simulink model "Copy_of_cd_barrowman_method"  (R2023a)
settings: Solver=VariableStepAuto  StartTime=0.0  StopTime=10.0  RelTol=1e-3
settings Model: Creator=aleco  LastModifiedBy=aleco

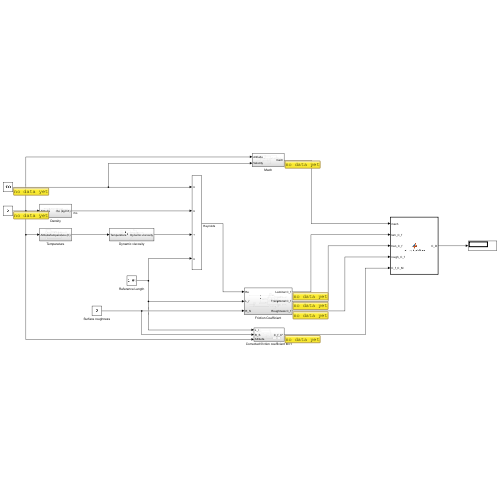
[thumbnail: Simulink's stored preview of the top-level diagram]
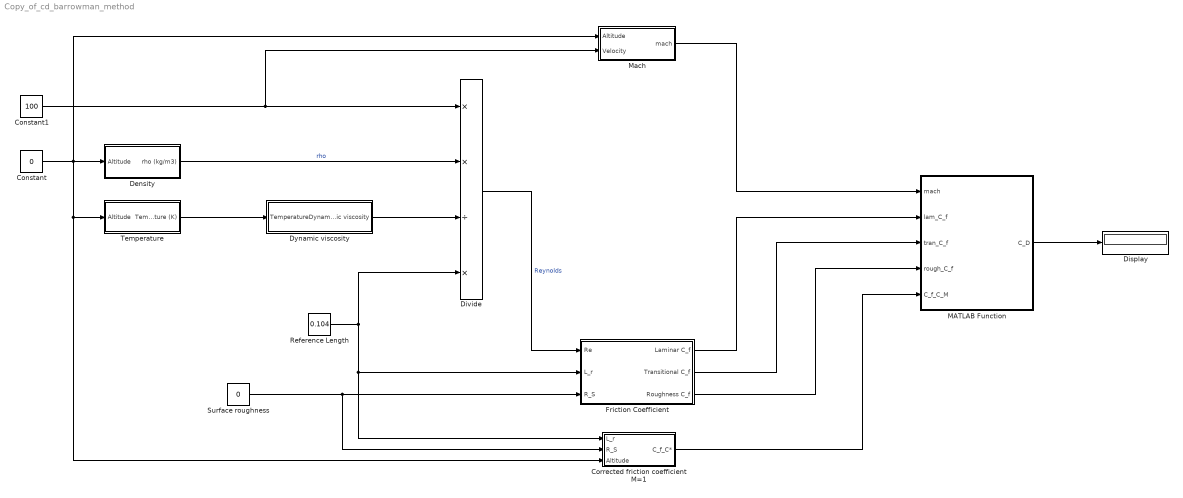
== system Copy_of_cd_barrowman_method ==
  Constant : Constant  Value=0
  Constant1 : Constant  Value=100
  Corrected friction coefficient M=1 : Subsystem
  Density : Subsystem
  Display : Display
  Divide : Product  Inputs=**/*
  Dynamic viscosity : Subsystem
  Friction Coefficient : Subsystem
  MATLAB Function : MATLAB Function  TreatAsAtomicUnit=on
  Mach : Subsystem
  Reference Length : Constant  Value=0.104
  Surface roughness : Constant  Value=0
  Temperature : Subsystem
  wires:
  Constant1/1 -> Divide/1, Mach/2(Velocity)
  Temperature/1(Temperature (K)) -> Dynamic viscosity/1(Temperature)
  Density/1(rho (kg/m3)) -> Divide/2  "rho"
  Reference Length/1 -> Divide/4, Corrected friction coefficient M=1/1(L_r), Friction Coefficient/2(L_r)
  Dynamic viscosity/1(Dynamic viscosity) -> Divide/3
  Surface roughness/1 -> Friction Coefficient/3(R_S), Corrected friction coefficient M=1/2(R_S)
  Divide/1 -> Friction Coefficient/1(Re)  "Reynolds"
  Constant/1 -> Mach/1(Altitude), Corrected friction coefficient M=1/3(Altitude), Temperature/1(Altitude), Density/1(Altitude)
  Mach/1(mach) -> MATLAB Function/1(mach)
  Friction Coefficient/1(Laminar C_f) -> MATLAB Function/2(lam_C_f)
  Friction Coefficient/2(Transitional C_f) -> MATLAB Function/3(tran_C_f)
  Friction Coefficient/3(Roughness C_f) -> MATLAB Function/4(rough_C_f)
  Corrected friction coefficient M=1/1(C_f_C*) -> MATLAB Function/5(C_f_C_M)
  MATLAB Function/1(C_D) -> Display/1

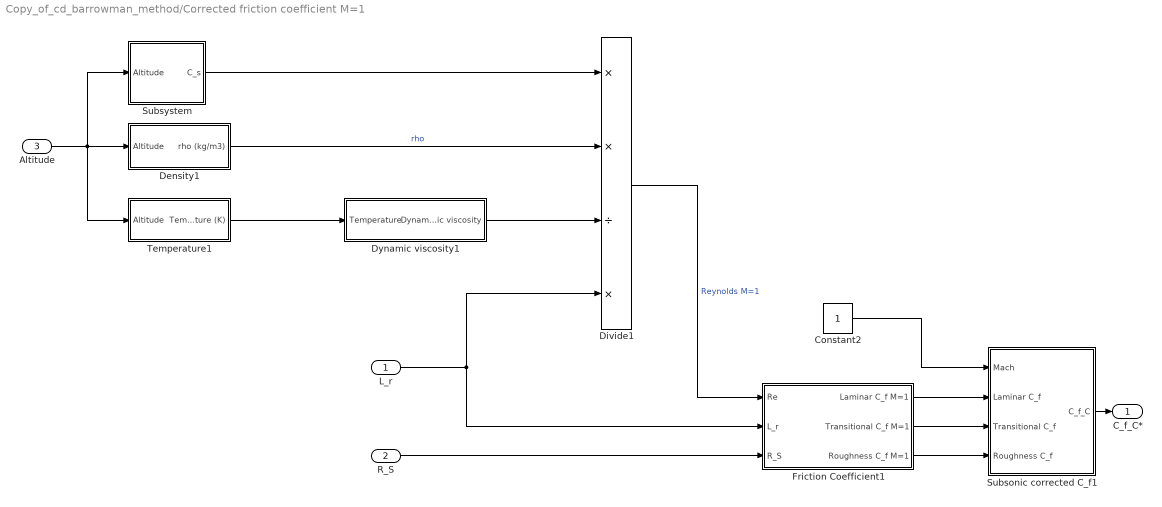
== system Copy_of_cd_barrowman_method/Corrected friction coefficient M=1 ==
  L_r : Inport
  R_S : Inport  Port=2
  Altitude : Inport  Port=3
  Constant2 : Constant
  Density1 : Subsystem
  Divide1 : Product  Inputs=**/*
  Dynamic viscosity1 : Subsystem
  Friction Coefficient1 : Subsystem
  Subsonic corrected C_f1 : Subsystem
  Subsystem : Subsystem
  Temperature1 : Subsystem
  C_f_C* : Outport
  wires:
  Temperature1/1(Temperature (K)) -> Dynamic viscosity1/1(Temperature)
  Subsystem/1(C_s) -> Divide1/1
  Divide1/1 -> Friction Coefficient1/1(Re)  "Reynolds M=1"
  R_S/1 -> Friction Coefficient1/3(R_S)
  Friction Coefficient1/1(Laminar C_f M=1) -> Subsonic corrected C_f1/2(Laminar C_f)
  L_r/1 -> Divide1/4, Friction Coefficient1/2(L_r)
  Friction Coefficient1/2(Transitional C_f M=1) -> Subsonic corrected C_f1/3(Transitional C_f)
  Friction Coefficient1/3(Roughness C_f M=1) -> Subsonic corrected C_f1/4(Roughness C_f)
  Dynamic viscosity1/1(Dynamic viscosity) -> Divide1/3
  Constant2/1 -> Subsonic corrected C_f1/1(Mach)
  Altitude/1 -> Subsystem/1(Altitude), Temperature1/1(Altitude), Density1/1(Altitude)
  Density1/1(rho (kg/m3)) -> Divide1/2  "rho"
  Subsonic corrected C_f1/1(C_f_C) -> C_f_C*/1

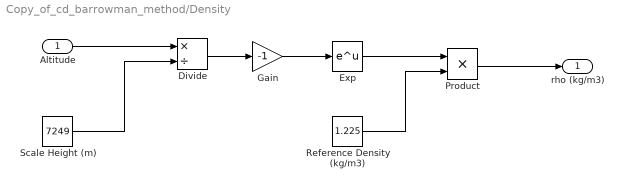
== system Copy_of_cd_barrowman_method/Density ==
  Altitude : Inport
  Divide : Product  Inputs=*/
  Exp : Math
  Gain : Gain  Gain=-1
  Product : Product
  Reference Density (kg/m3) : Constant  Value=1.225
  Scale Height (m) : Constant  Value=7249
  rho (kg/m3) : Outport
  wires:
  Altitude/1 -> Divide/1
  Scale Height (m)/1 -> Divide/2
  Divide/1 -> Gain/1
  Gain/1 -> Exp/1
  Exp/1 -> Product/1
  Reference Density (kg/m3)/1 -> Product/2
  Product/1 -> rho (kg/m3)/1

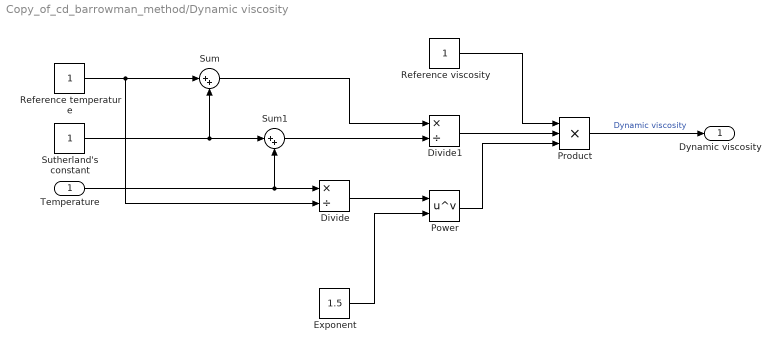
== system Copy_of_cd_barrowman_method/Dynamic viscosity ==
  Temperature : Inport
  Divide : Product  Inputs=*/
  Divide1 : Product  Inputs=*/
  Exponent : Constant  Value=1.5
  Power : Math  Operator=pow
  Product : Product  Inputs=3
  Reference temperature : Constant
  Reference viscosity : Constant
  Sum : Sum  Inputs=|++
  Sum1 : Sum  Inputs=|++
  Sutherland's constant : Constant
  Dynamic viscosity : Outport
  wires:
  Sum/1 -> Divide1/1
  Divide/1 -> Power/1
  Temperature/1 -> Sum1/2, Divide/1
  Sutherland's constant/1 -> Sum/2, Sum1/1
  Reference temperature/1 -> Divide/2, Sum/1
  Sum1/1 -> Divide1/2
  Exponent/1 -> Power/2
  Divide1/1 -> Product/2
  Product/1 -> Dynamic viscosity/1  "Dynamic viscosity"
  Reference viscosity/1 -> Product/1
  Power/1 -> Product/3

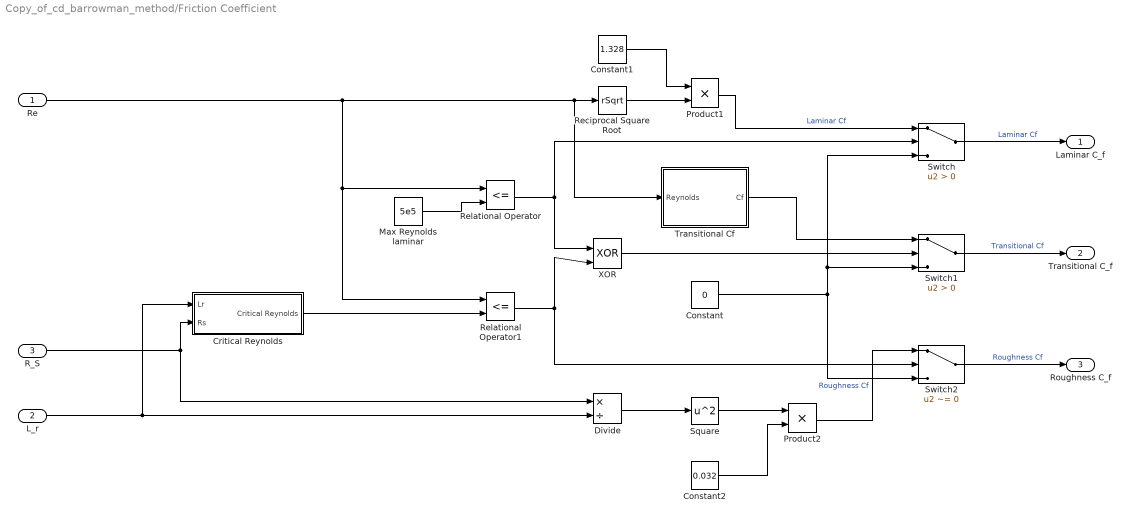
== system Copy_of_cd_barrowman_method/Friction Coefficient ==
  Re : Inport
  L_r : Inport  Port=2
  R_S : Inport  Port=3
  Constant : Constant  Value=0
  Constant1 : Constant  Value=1.328
  Constant2 : Constant  Value=0.032
  Critical Reynolds : Subsystem
  Divide : Product  Inputs=*/
  Max Reynolds laminar : Constant  Value=5e5
  Product1 : Product
  Product2 : Product
  Reciprocal Square Root : Sqrt  Operator=rSqrt
  Relational Operator : RelationalOperator  Operator=<=  OutDataTypeStr=boolean  RndMeth=Simplest  InputSameDT=off
  Relational Operator1 : RelationalOperator  Operator=<=  OutDataTypeStr=boolean  RndMeth=Simplest  InputSameDT=off
  Square : Math  Operator=square
  Switch : Switch  Criteria=u2 > Threshold  SaturateOnIntegerOverflow=off  InputSameDT=off
  Switch1 : Switch  Criteria=u2 > Threshold  SaturateOnIntegerOverflow=off  InputSameDT=off
  Switch2 : Switch  Criteria=u2 ~= 0  SaturateOnIntegerOverflow=off  InputSameDT=off
  Transitional Cf : Subsystem
  XOR : Logic  Operator=XOR  IconShape=distinctive  AllPortsSameDT=off  OutDataTypeStr=boolean
  Laminar C_f : Outport
  Transitional C_f : Outport  Port=2
  Roughness C_f : Outport  Port=3
  wires:
  Constant/1 -> Switch/3, Switch1/3, Switch2/3
  Reciprocal Square Root/1 -> Product1/2
  Transitional Cf/1(Cf) -> Switch1/1
  Switch2/1 -> Roughness C_f/1  "Roughness Cf"
  Product1/1 -> Switch/1  "Laminar Cf"
  Critical Reynolds/1(Critical Reynolds) -> Relational Operator1/2
  Relational Operator1/1 -> Switch2/2, XOR/2
  Re/1 -> Transitional Cf/1(Reynolds), Reciprocal Square Root/1, Relational Operator/1, Relational Operator1/1
  Product2/1 -> Switch2/1  "Roughness Cf"
  XOR/1 -> Switch1/2
  R_S/1 -> Critical Reynolds/2(Rs), Divide/1
  Constant1/1 -> Product1/1
  Switch1/1 -> Transitional C_f/1  "Transitional Cf"
  L_r/1 -> Critical Reynolds/1(Lr), Divide/2
  Relational Operator/1 -> Switch/2, XOR/1
  Max Reynolds laminar/1 -> Relational Operator/2
  Divide/1 -> Square/1
  Switch/1 -> Laminar C_f/1  "Laminar Cf"
  Square/1 -> Product2/1
  Constant2/1 -> Product2/2

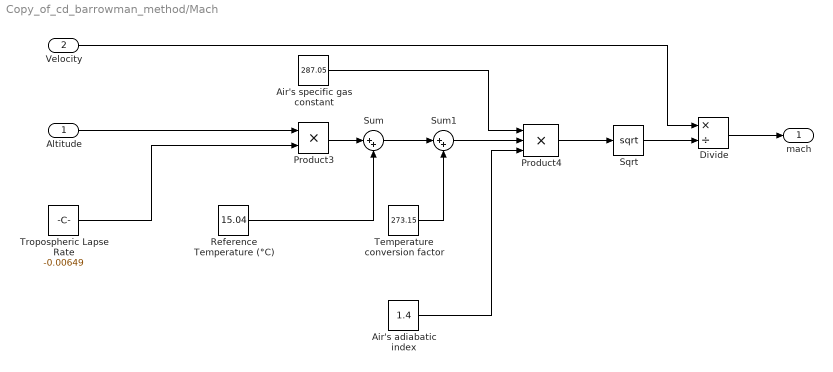
== system Copy_of_cd_barrowman_method/Mach ==
  Altitude : Inport
  Velocity : Inport  Port=2
  Air's adiabatic index : Constant  Value=1.4
  Air's specific gas constant : Constant  Value=287.05
  Divide : Product  Inputs=*/
  Product3 : Product
  Product4 : Product  Inputs=3
  Reference Temperature (°C) : Constant  Value=15.04
  Sqrt : Sqrt
  Sum : Sum  Inputs=|++
  Sum1 : Sum  Inputs=|++
  Temperature conversion factor : Constant  Value=273.15
  Tropospheric Lapse Rate : Constant  Value=-0.00649
  mach : Outport
  wires:
  Product4/1 -> Sqrt/1
  Product3/1 -> Sum/1
  Air's adiabatic index/1 -> Product4/3
  Tropospheric Lapse Rate/1 -> Product3/2
  Air's specific gas constant/1 -> Product4/1
  Sum/1 -> Sum1/1
  Reference Temperature (°C)/1 -> Sum/2
  Altitude/1 -> Product3/1
  Velocity/1 -> Divide/1
  Divide/1 -> mach/1
  Temperature conversion factor/1 -> Sum1/2
  Sum1/1 -> Product4/2
  Sqrt/1 -> Divide/2

== system Copy_of_cd_barrowman_method/Temperature ==
  Altitude : Inport
  Factor of conversion to K : Constant  Value=273.15
  Product3 : Product
  Reference Temperature (°C) : Constant  Value=15.04
  Sum : Sum  Inputs=|++
  Sum1 : Sum  Inputs=|++
  Tropospheric Lapse Rate : Constant  Value=-0.00649
  Temperature (K) : Outport
  wires:
  Altitude/1 -> Product3/1
  Sum/1 -> Sum1/1
  Tropospheric Lapse Rate/1 -> Product3/2
  Product3/1 -> Sum/1
  Factor of conversion to K/1 -> Sum1/2
  Sum1/1 -> Temperature (K)/1
  Reference Temperature (°C)/1 -> Sum/2

== system Copy_of_cd_barrowman_method/Corrected friction coefficient M=1/Density1 ==
  Altitude : Inport
  Divide : Product  Inputs=*/
  Exp : Math
  Gain : Gain  Gain=-1
  Product : Product
  Reference Density (kg/m3) : Constant  Value=1.225
  Scale Height (m) : Constant  Value=7249
  rho (kg/m3) : Outport
  wires:
  Altitude/1 -> Divide/1
  Scale Height (m)/1 -> Divide/2
  Divide/1 -> Gain/1
  Gain/1 -> Exp/1
  Exp/1 -> Product/1
  Reference Density (kg/m3)/1 -> Product/2
  Product/1 -> rho (kg/m3)/1

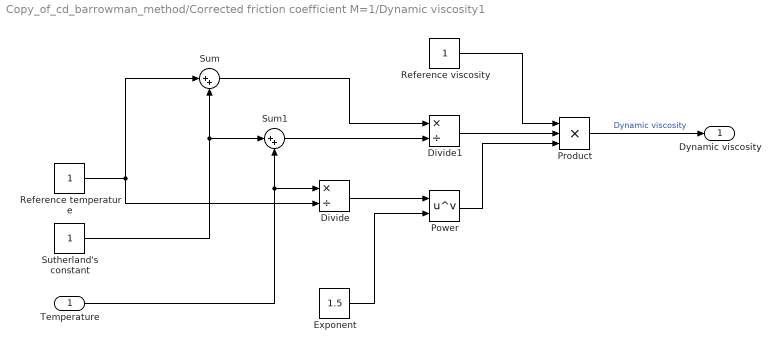
== system Copy_of_cd_barrowman_method/Corrected friction coefficient M=1/Dynamic viscosity1 ==
  Temperature : Inport
  Divide : Product  Inputs=*/
  Divide1 : Product  Inputs=*/
  Exponent : Constant  Value=1.5
  Power : Math  Operator=pow
  Product : Product  Inputs=3
  Reference temperature : Constant
  Reference viscosity : Constant
  Sum : Sum  Inputs=|++
  Sum1 : Sum  Inputs=|++
  Sutherland's constant : Constant
  Dynamic viscosity : Outport
  wires:
  Sum/1 -> Divide1/1
  Divide/1 -> Power/1
  Temperature/1 -> Sum1/2, Divide/1
  Sutherland's constant/1 -> Sum/2, Sum1/1
  Reference temperature/1 -> Divide/2, Sum/1
  Sum1/1 -> Divide1/2
  Exponent/1 -> Power/2
  Divide1/1 -> Product/2
  Product/1 -> Dynamic viscosity/1  "Dynamic viscosity"
  Reference viscosity/1 -> Product/1
  Power/1 -> Product/3

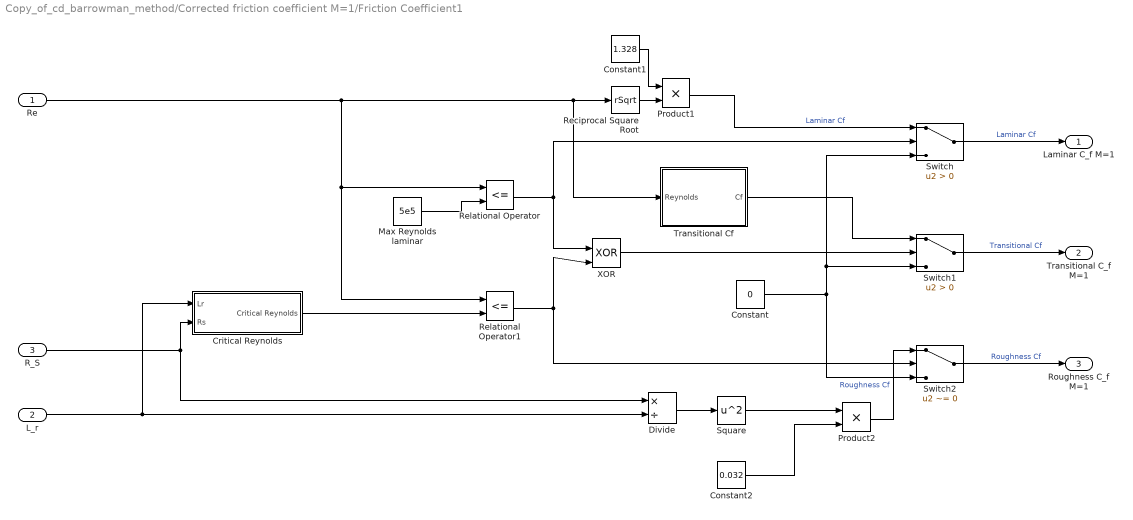
== system Copy_of_cd_barrowman_method/Corrected friction coefficient M=1/Friction Coefficient1 ==
  Re : Inport
  L_r : Inport  Port=2
  R_S : Inport  Port=3
  Constant : Constant  Value=0
  Constant1 : Constant  Value=1.328
  Constant2 : Constant  Value=0.032
  Critical Reynolds : Subsystem
  Divide : Product  Inputs=*/
  Max Reynolds laminar : Constant  Value=5e5
  Product1 : Product
  Product2 : Product
  Reciprocal Square Root : Sqrt  Operator=rSqrt
  Relational Operator : RelationalOperator  Operator=<=  OutDataTypeStr=boolean  RndMeth=Simplest  InputSameDT=off
  Relational Operator1 : RelationalOperator  Operator=<=  OutDataTypeStr=boolean  RndMeth=Simplest  InputSameDT=off
  Square : Math  Operator=square
  Switch : Switch  Criteria=u2 > Threshold  SaturateOnIntegerOverflow=off  InputSameDT=off
  Switch1 : Switch  Criteria=u2 > Threshold  SaturateOnIntegerOverflow=off  InputSameDT=off
  Switch2 : Switch  Criteria=u2 ~= 0  SaturateOnIntegerOverflow=off  InputSameDT=off
  Transitional Cf : Subsystem
  XOR : Logic  Operator=XOR  IconShape=distinctive  AllPortsSameDT=off  OutDataTypeStr=boolean
  Laminar C_f M=1 : Outport
  Transitional C_f M=1 : Outport  Port=2
  Roughness C_f M=1 : Outport  Port=3
  wires:
  Constant/1 -> Switch/3, Switch1/3, Switch2/3
  Reciprocal Square Root/1 -> Product1/2
  Transitional Cf/1(Cf) -> Switch1/1
  Switch2/1 -> Roughness C_f M=1/1  "Roughness Cf"
  Product1/1 -> Switch/1  "Laminar Cf"
  Critical Reynolds/1(Critical Reynolds) -> Relational Operator1/2
  Relational Operator1/1 -> Switch2/2, XOR/2
  Re/1 -> Transitional Cf/1(Reynolds), Reciprocal Square Root/1, Relational Operator/1, Relational Operator1/1
  Product2/1 -> Switch2/1  "Roughness Cf"
  XOR/1 -> Switch1/2
  R_S/1 -> Critical Reynolds/2(Rs), Divide/1
  Constant1/1 -> Product1/1
  Switch1/1 -> Transitional C_f M=1/1  "Transitional Cf"
  L_r/1 -> Critical Reynolds/1(Lr), Divide/2
  Relational Operator/1 -> Switch/2, XOR/1
  Max Reynolds laminar/1 -> Relational Operator/2
  Divide/1 -> Square/1
  Switch/1 -> Laminar C_f M=1/1  "Laminar Cf"
  Square/1 -> Product2/1
  Constant2/1 -> Product2/2

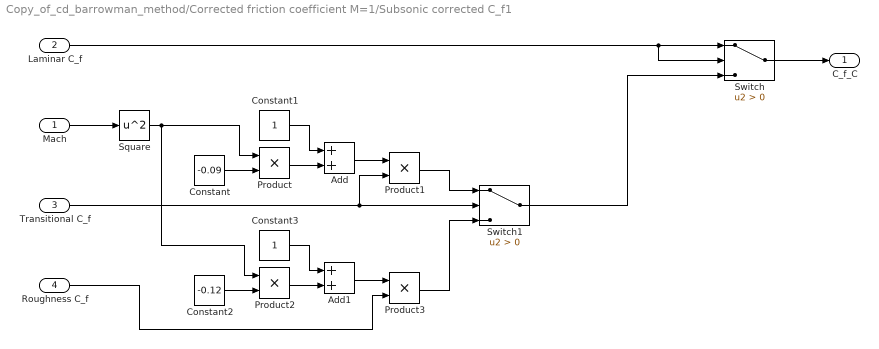
== system Copy_of_cd_barrowman_method/Corrected friction coefficient M=1/Subsonic corrected C_f1 ==
  Mach : Inport
  Laminar C_f : Inport  Port=2
  Transitional C_f : Inport  Port=3
  Roughness C_f : Inport  Port=4
  Add : Sum
  Add1 : Sum
  Constant : Constant  Value=-0.09
  Constant1 : Constant
  Constant2 : Constant  Value=-0.12
  Constant3 : Constant
  Product{,1..3} (4 alike) : Product
  Square : Math  Operator=square
  Switch : Switch  Criteria=u2 > Threshold  SaturateOnIntegerOverflow=off  InputSameDT=off
  Switch1 : Switch  Criteria=u2 > Threshold  SaturateOnIntegerOverflow=off  InputSameDT=off
  C_f_C : Outport
  wires:
  Laminar C_f/1 -> Switch/2, Switch/1
  Switch/1 -> C_f_C/1
  Transitional C_f/1 -> Product1/2, Switch1/2
  Mach/1 -> Square/1
  Constant/1 -> Product/2
  Square/1 -> Product2/1, Product/1
  Constant1/1 -> Add/1
  Product/1 -> Add/2
  Add/1 -> Product1/1
  Product1/1 -> Switch1/1
  Switch1/1 -> Switch/3
  Constant2/1 -> Product2/2
  Add1/1 -> Product3/1
  Product2/1 -> Add1/2
  Constant3/1 -> Add1/1
  Roughness C_f/1 -> Product3/2
  Product3/1 -> Switch1/3

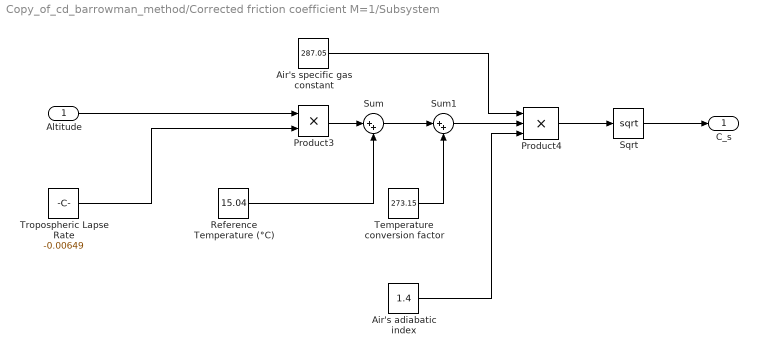
== system Copy_of_cd_barrowman_method/Corrected friction coefficient M=1/Subsystem ==
  Altitude : Inport
  Air's adiabatic index : Constant  Value=1.4
  Air's specific gas constant : Constant  Value=287.05
  Product3 : Product
  Product4 : Product  Inputs=3
  Reference Temperature (°C) : Constant  Value=15.04
  Sqrt : Sqrt
  Sum : Sum  Inputs=|++
  Sum1 : Sum  Inputs=|++
  Temperature conversion factor : Constant  Value=273.15
  Tropospheric Lapse Rate : Constant  Value=-0.00649
  C_s : Outport
  wires:
  Sum/1 -> Sum1/1
  Air's specific gas constant/1 -> Product4/1
  Air's adiabatic index/1 -> Product4/3
  Sum1/1 -> Product4/2
  Product4/1 -> Sqrt/1
  Temperature conversion factor/1 -> Sum1/2
  Tropospheric Lapse Rate/1 -> Product3/2
  Product3/1 -> Sum/1
  Reference Temperature (°C)/1 -> Sum/2
  Altitude/1 -> Product3/1
  Sqrt/1 -> C_s/1

== system Copy_of_cd_barrowman_method/Corrected friction coefficient M=1/Temperature1 ==
  Altitude : Inport
  Factor of conversion to K : Constant  Value=273.15
  Product3 : Product
  Reference Temperature (°C) : Constant  Value=15.04
  Sum : Sum  Inputs=|++
  Sum1 : Sum  Inputs=|++
  Tropospheric Lapse Rate : Constant  Value=-0.00649
  Temperature (K) : Outport
  wires:
  Altitude/1 -> Product3/1
  Sum/1 -> Sum1/1
  Tropospheric Lapse Rate/1 -> Product3/2
  Product3/1 -> Sum/1
  Factor of conversion to K/1 -> Sum1/2
  Sum1/1 -> Temperature (K)/1
  Reference Temperature (°C)/1 -> Sum/2

== system Copy_of_cd_barrowman_method/Friction Coefficient/Critical Reynolds ==
  Lr : Inport
  Rs : Inport  Port=2
  Constant : Constant  Value=51
  Constant1 : Constant  Value=-1.039
  Divide : Product  Inputs=*/
  Power : Math  Operator=pow
  Product1 : Product
  Critical Reynolds : Outport
  wires:
  Divide/1 -> Power/1
  Power/1 -> Product1/1
  Constant1/1 -> Power/2
  Constant/1 -> Product1/2
  Product1/1 -> Critical Reynolds/1  "Critical Reynolds"
  Lr/1 -> Divide/2
  Rs/1 -> Divide/1

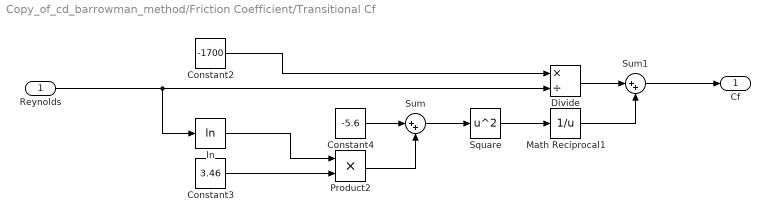
== system Copy_of_cd_barrowman_method/Friction Coefficient/Transitional Cf ==
  Reynolds : Inport
  Constant2 : Constant  Value=-1700
  Constant3 : Constant  Value=3.46
  Constant4 : Constant  Value=-5.6
  Divide : Product  Inputs=*/
  Math Reciprocal1 : Math  Operator=reciprocal  SignedPower=on
  Product2 : Product
  Square : Math  Operator=square
  Sum : Sum  Inputs=|++
  Sum1 : Sum  Inputs=|++
  ln : Math  Operator=log
  Cf : Outport
  wires:
  Math Reciprocal1/1 -> Sum1/2
  Constant2/1 -> Divide/1
  Product2/1 -> Sum/2
  Reynolds/1 -> ln/1, Divide/2
  Square/1 -> Math Reciprocal1/1
  Constant4/1 -> Sum/1
  Divide/1 -> Sum1/1
  ln/1 -> Product2/1
  Constant3/1 -> Product2/2
  Sum/1 -> Square/1
  Sum1/1 -> Cf/1

== system Copy_of_cd_barrowman_method/Corrected friction coefficient M=1/Friction Coefficient1/Critical Reynolds ==
  Lr : Inport
  Rs : Inport  Port=2
  Constant : Constant  Value=51
  Constant1 : Constant  Value=-1.039
  Divide : Product  Inputs=*/
  Power : Math  Operator=pow
  Product1 : Product
  Critical Reynolds : Outport
  wires:
  Divide/1 -> Power/1
  Power/1 -> Product1/1
  Constant1/1 -> Power/2
  Constant/1 -> Product1/2
  Product1/1 -> Critical Reynolds/1  "Critical Reynolds"
  Lr/1 -> Divide/2
  Rs/1 -> Divide/1

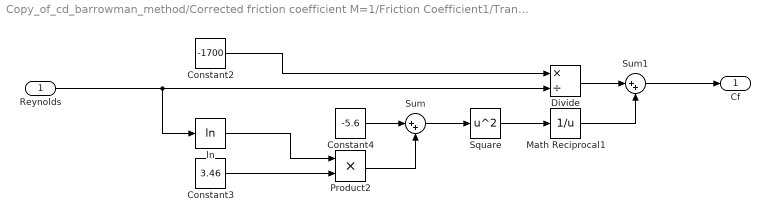
== system Copy_of_cd_barrowman_method/Corrected friction coefficient M=1/Friction Coefficient1/Transitional Cf ==
  Reynolds : Inport
  Constant2 : Constant  Value=-1700
  Constant3 : Constant  Value=3.46
  Constant4 : Constant  Value=-5.6
  Divide : Product  Inputs=*/
  Math Reciprocal1 : Math  Operator=reciprocal  SignedPower=on
  Product2 : Product
  Square : Math  Operator=square
  Sum : Sum  Inputs=|++
  Sum1 : Sum  Inputs=|++
  ln : Math  Operator=log
  Cf : Outport
  wires:
  Math Reciprocal1/1 -> Sum1/2
  Constant2/1 -> Divide/1
  Product2/1 -> Sum/2
  Reynolds/1 -> ln/1, Divide/2
  Square/1 -> Math Reciprocal1/1
  Constant4/1 -> Sum/1
  Divide/1 -> Sum1/1
  ln/1 -> Product2/1
  Constant3/1 -> Product2/2
  Sum/1 -> Square/1
  Sum1/1 -> Cf/1

== matlab function Copy_of_cd_barrowman_method/MATLAB Function ==
  data: mach input; C_D output; lam_C_f input; tran_C_f input; rough_C_f input; C_f_C_M input
function C_D = cd_calculation(mach,lam_C_f,tran_C_f,rough_C_f,C_f_C_M)
% %% SETUP OF THE ROCKET'S GEOMETRY
% N = 4; % number of fins
% A_T = 0.0135; % planform area of a single fin
% A_r = 0.008495; % reference area
% f_b = 20.77; % fineness ratio of the body
% A_W_B = 1.245; % total wetted area of the body
% S = 0.1; % fin's span
% gamma_L = pi/4; % leading edge sweepback angle
% r_L = 0.002; % radius of the rounded leading edge
% c_r = 0.2; % fin's root chord
% h_r = 0.004; % root trailing edge thickness of the fin
% t_r = 0.05; % maximum thickness of the fin
% gamma_C = 0.994; % midcord line sweepback angle
% A_B_f = 9e-3; % fin's base area
% f_n = 5; % fineness ratio of the nose
% A_B = 0.008495; % base area
% %% C_D CALCULATION
% if mach^2 <= 0.1 %incompressible flow
%     %% COEFFICIENT OF FRICTION
%     C_f = lam_C_f + tran_C_f + rough_C_f; % adding the C_f directly as just
%     % one of them will be different than zero
%     %% FRICTION DRAG COEFFICIENT
%     C_D_f_t = 2 * N * C_f * A_T * A_r; % tail
%     C_D_f_b = (1 + (0.5 / f_b)) * C_f * A_W_B / A_r; % body
%     C_D_f = C_D_f_b + C_D_f_t; % friction drag coefficient
%     %% FINS' DRAG COEFFICIENTS
%     delta_C_D = ((1 - mach^2)^-0.417) - 1;
%     C_D_L_T = 2 * N * S * r_L * cos(gamma_L)^2 * delta_C_D / A_r; % leading
%     % edge pressure drag
%     C_f_B = 2 * C_f * c_r / h_r;
%     C_D_B_T = 0.135 * N / (C_f_B^(1/3)); % trailing edge base drag
%     AR = S^2 / A_T; % aspect ratio of the fin
%     epsilon = AR * t_r^(1/3) / c_r;
%     C_D_TT_M = 1.15 * (t_r / c_r)^(5/3) * (1.61 + epsilon - ...
%         sqrt((epsilon - 1.43)^2 + 0.578));
%     K = cos(gamma_C)^2 + ((C_D_TT_M * A_r / (C_f_C_M * A_T) - ...
%         4 * t_r * cos(gamma_C) / c_r) / ...
%         (120 * (t_r / c_r)^4 * cos(gamma_C)^2));% prandtl correcting factor
%     C_D_TT = 4 * N * C_f * (A_T / A_r) * (t_r * cos(gamma_C) / c_r + ...
%         30 * (t_r / c_r)^4 * cos(gamma_C)^2 / ...
%         ((K - mach^2 * cos(gamma_C)^2)^(3/2)));% thickness pressure drag
%     % coefficient
%     %% BODY'S DRAG COEFFICIENTS
%     K_og = 1 + (6.82 * A_W_B * C_f_C_M * (f_n + 1)^2.22 / (f_b^3 * A_r));
%     % ogive
%     C_D_P = 6 * A_W_B * C_f / (f_b^3 * A_r * (K_og - mach^2)^0.6);% body
%     % pressure drag
%     C_D_B = 0.029 / sqrt(C_f * A_W_B / A_B); % body base drag
%     %% TOTAL DRAG COEFFICIENT
%     C_D = C_D_f + C_D_L_T + C_D_B_T + C_D_TT + C_D_P + C_D_B;
% elseif mach <= 1 %subsonic flow
%     %% CORRECTED COEFFICIENT OF FRICTION
%     if lam_C_f ~= 0
%         C_f_C = lam_C_f;
%     elseif tran_C_f ~= 0
%         C_f_C = tran_C_f * (1 - 0.09 * mach^2);
%     else
%         C_f_C = rough_C_f * (1 - 0.12 * mach^2);
%     end
%     %% FRICTION DRAG COEFFICIENT
%     C_D_f_t = 2 * N * C_f_C * A_T * A_r; % tail
%     C_D_f_b = (1 + (0.5/f_b)) * C_f_C * A_W_B / A_r; % body
%     C_D_f = C_D_f_b + C_D_f_t; % friction drag coefficient
%     %% FINS' DRAG COEFFICIENTS
%     if mach < 0.9
%         delta_C_D = ((1 - mach^2)^-0.417) - 1;
%     else
%         delta_C_D = 1 - 1.5 * (mach - 0.9);
%     end
%     C_D_L_T = 2 * N * S * r_L * cos(gamma_L)^2 * delta_C_D / A_r; % leading
%     % edge pressure drag
%     C_f_B = 2 * C_f_C * c_r / h_r;
%     K_1 = cos(gamma_C)^2 + (0.223 + 4.02 * C_f_C_M * (t_r / h_r)^2)^2 / ...
%         (c_r * C_f_C_M * h_r)^(2/3); % prandtl correcting factor
%     C_D_B_T = 0.135 * N * A_B_f / (A_r * C_f_B^(1/3) * ...
%         sqrt(K_1 - mach^2 * cos(gamma_C)^2)); % trailing edge base drag
%     AR = S^2 / A_T; % aspect ratio of the fin
%     epsilon = AR * t_r^(1/3) / c_r;
%     C_D_TT_M = 1.15 * (t_r / c_r)^(5/3) * (1.61 + epsilon - ...
%         sqrt((epsilon - 1.43)^2 + 0.578));
%     K_2 = cos(gamma_C)^2 + ((C_D_TT_M * A_r / (C_f_C_M * A_T) - ...
%         4 * t_r * cos(gamma_C) / c_r) / ...
%         (120 * (t_r / c_r)^4 * cos(gamma_C)^2));% prandtl correcting factor
%     C_D_TT = 4 * N * C_f_C * (A_T / A_r) * (t_r * cos(gamma_C) / c_r + ...
%         30 * (t_r / c_r)^4 * cos(gamma_C)^2 / ...
%         ((K_2 - mach^2 * cos(gamma_C)^2)^(3/2)));% thickness pressure drag
%     % coefficient
%     %% BODY'S DRAG COEFFICIENTS
%     K_og = 1 + (6.82 * A_W_B * C_f_C_M * (f_n + 1)^2.22 / (f_b^3 * A_r));
%     % ogive
%     C_D_P = 6 * A_W_B * C_f_C / (f_b^3 * A_r * (K_og - mach^2)^0.6);% body
%     % pressure drag
%     K_3 = 1 + A_B / ((6.38 + 39.7 * h_r / c_r) * C_f_C_M * A_W_B);% prandtl
%     % correcting factor
%     C_D_B = 0.029 * A_B / ...
%         (A_r * sqrt(C_f_C * A_W_B * (K_3 - mach^2) / A_B));
%     %% TOTAL DRAG COEFFICIENT
%     C_D = C_D_f + C_D_L_T + C_D_B_T + C_D_TT + C_D_P + C_D_B;
% else %supersonic flow
%     %% CORRECTED COEFFICIENT OF FRICTION
%     if lam_C_f ~= 0
%         C_f_C = lam_C_f / ((1 + 0.045 *mach^2)^0.25);
%     elseif tran_C_f ~= 0
%         C_f_C = tran_C_f / ((1 + 0.15 *mach^2)^0.58); % with K = 0.15
%     else
%         C_f_C = rough_C_f / (1 + 0.18 *mach^2);
%     end
%     %% FRICTION DRAG COEFFICIENT
%     C_D_f_t = 2 * N * C_f_C * A_T * A_r; % tail
%     C_D_f_b = (1 + (0.5 / f_b)) * C_f_C * A_W_B / A_r; % body
%     C_D_f = C_D_f_b + C_D_f_t; % friction drag coefficient
%     %% FINS' DRAG COEFFICIENTS
%     delta_C_D = 1.214 - (0.502 / (mach^2)) + (0.1095 / (mach^4)) + ...
%         (0.0231 / (mach^6));
%     C_D_L_T = 2 * N * S * r_L * cos(gamma_L)^2 * delta_C_D / A_r; % leading
%     % edge pressure drag
%     C_D_B_T = N * (1 - 0.52 * mach^-1.19) * A_B_f / ...
%         (A_r * (1 + 18 * C_f_C_M * (t_r / h_r)^2) * mach^2); % trailing
%     % edge base drag
%     %
%     %% ADD HERE WAVE DRAG CALCULATION FOR THE FINS
%     %
%     %% BODY'S DRAG COEFFICIENTS
%     %
%     %% ADD HERE BODY PRESSURE DRAG CALCULATION
%     %
%     C_D_B_M = A_B * (0.185 + 1.15 * (h_r / c_r)) / A_r;
%     M_cr = 0.892 * sqrt(C_D_B_M);
%     if mach <= M_cr
%         C_D_B = C_D_B_M * (0.88 + 0.12 * exp(-3.58 * (mach - 1)));
%     else
%         C_D_B = 0.7 * A_B / (A_r * mach^2);
%     end
%     %% TOTAL DRAG COEFFICIENT
%     C_D = C_D_f + C_D_L_T + C_D_B_T + C_D_B; % wave drag and body pressure
%     % drag contributions are missing
C_D = 1;
end
